simulink model "Progetto_Gruppo21_IZ"  (R2024b)
settings: Solver=FixedStepDiscrete  StartTime=0.0  StopTime=300  FixedStep=0.5  RelTol=1e-3  EnableMultiTasking=on
(part 1 of 2)
settings Model: PacingRate=0.500000  Creator=angel  LastModifiedBy=angel
settings OptimizationCC: DefaultParameterBehavior=Inlined  EnhancedBackFolding=on  PassReuseOutputArgsAs=Individual arguments  ZeroExternalMemoryAtStartup=off  ZeroInternalMemoryAtStartup=off  MaxStackSize=512  OptimizeBlockOrder=speed  DifferentSizesBufferReuse=on  OptimizationCustomize=off  EfficientTunableParamExpr=on
settings DebuggingCC: ParameterTunabilityLossMsg=error
settings HardwareCC: ProdBitPerPointer=32  ProdBitPerSizeT=32  ProdBitPerPtrDiffT=32  ProdLargestAtomicInteger=Long  ProdLargestAtomicFloat=Double  ProdWordSize=32  ProdLongLongMode=on  ProdHWDeviceType=ARM Compatible->ARM Cortex-M
settings RTWCC: Description=Embedded Coder  SystemTargetFile=ert.tlc  HardwareBoard=STM32G4xx Based  TemplateMakefile=ert_default_tmf  Toolchain=GNU Tools for ARM Embedded Processors
settings CodeAppCC: ForceParamTrailComments=on  IgnoreCustomStorageClasses=off  OperatorAnnotations=on  SimulinkDataObjDesc=on  SFDataObjDesc=on  InsertBlockDesc=on
settings ERTTargetCC: TargetLangStandard=C99 (ISO)  CodeReplacementLibrary=ARM Cortex-M  SupportVariableSizeSignals=on  ExtModeTransport=3  ExtModeStaticAlloc=on  ExtModeStaticAllocSize=2048  ExtModeMexFile=ext_xcp  ExtModeIntrfLevel=Level2 - Open

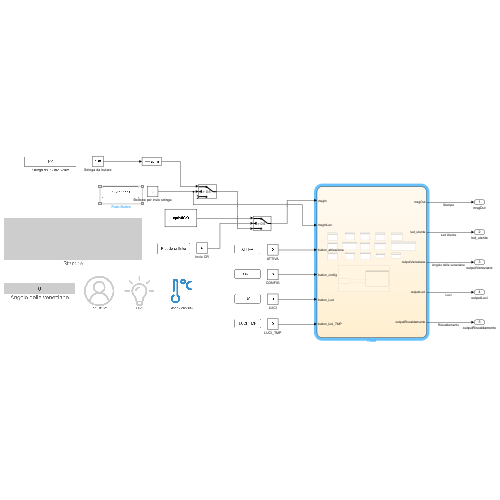
[thumbnail: Simulink's stored preview of the top-level diagram]
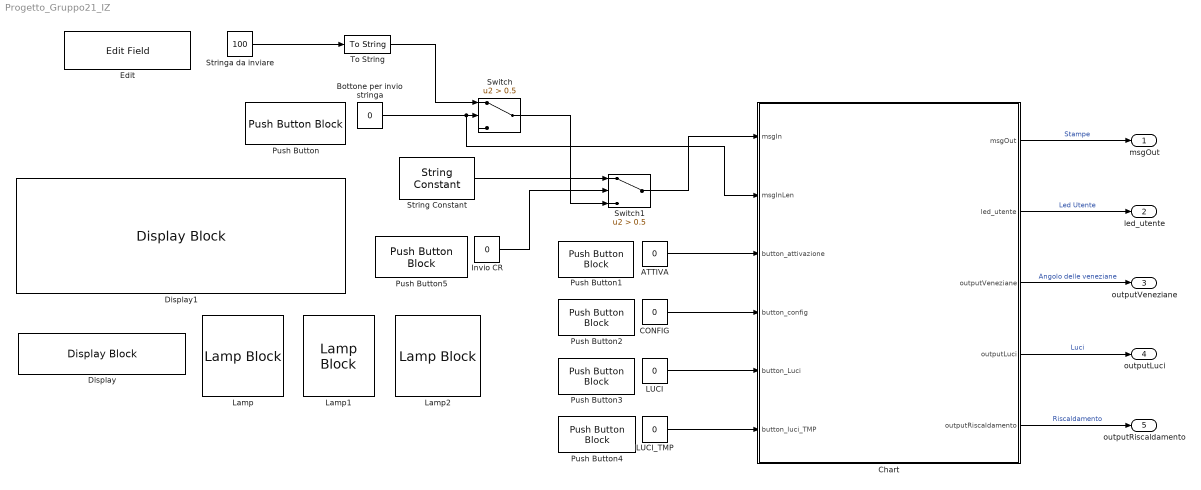
== system Progetto_Gruppo21_IZ ==
  ATTIVA : Constant  Value=0
  Bottone per invio stringa : Constant  Value=0
  CONFIG : Constant  Value=0
  Chart : Stateflow chart  TreatAsAtomicUnit=on
  Display : DisplayBlock  LabelPosition=Bottom  Transparency=1
  Display1 : DisplayBlock  LabelPosition=Bottom  Alignment=Left  Transparency=1
  Edit : EditField  LabelPosition=Bottom  ShowInitialText=on  Alignment=Center
  Invio CR : Constant  Value=0
  LUCI : Constant  Value=0
  LUCI_TMP : Constant  Value=0
  Lamp : LampBlock  LabelPosition=Bottom  Icon=Custom  CustomIcon=data:image/svg+xml;base64,CjwhLS0gR2VuZXJhdG9yOiB2aXNpb25jb3J0ZXggVlRyYWNlciAwLjYuNCAtLT4KPHN2ZyB2ZXJzaW9uPSIxLjEiIHhtbG5zPSJodHRwOi8vd3d3LnczLm9yZy8yMDAwL3N2ZyIgdmlld0JveD0iMCAwIDUxMiA1MTIiIHByZXNlcnZlQXNwZWN0UmF0aW89InhNaWRZTWlkIG1lZXQiPgo8cGF0aCBkPSJNMCAwIEMwLjk2NyAwLjAwMiAxLjkzNSAwLjAwNCAyLjkzMSAwLjAwNiBDMTcuMjY0IDAuMDUxIDMxLjIxIDAuNTYgNDUuMzEyIDMuMzEyIEM0Ni42NTggMy41NTQgNDYuNjU4IDMuNTU0IDQ4LjAzMSAzLjggQzk2LjcxOCAxMi42 ...(+8728 chars)
  Lamp1 : LampBlock  LabelPosition=Bottom  Icon=Custom  CustomIcon=data:image/svg+xml;base64,CjwhLS0gR2VuZXJhdG9yOiB2aXNpb25jb3J0ZXggVlRyYWNlciAwLjYuNCAtLT4KPHN2ZyB2ZXJzaW9uPSIxLjEiIHhtbG5zPSJodHRwOi8vd3d3LnczLm9yZy8yMDAwL3N2ZyIgdmlld0JveD0iMCAwIDUxMiA1MTIiIHByZXNlcnZlQXNwZWN0UmF0aW89InhNaWRZTWlkIG1lZXQiPgo8cGF0aCBkPSJNMCAwIEMwLjY2NSAwLjE4MiAxLjMzMSAwLjM2NCAyLjAxNyAwLjU1MSBDMjQuMjc0IDYuNzU2IDQzLjIzNiAxOS40MzkgNjAgMzUgQzYwLjY1NiAzNS41NzkgNjEuMzEyIDM2LjE1OCA2MS45ODggMzYuNzU0IEM4Mi4yNjEgNTUu ...(+12092 chars)
  Lamp2 : LampBlock  LabelPosition=Bottom  Icon=Custom  CustomIcon=data:image/svg+xml;base64,CjwhLS0gR2VuZXJhdG9yOiB2aXNpb25jb3J0ZXggVlRyYWNlciAwLjYuNCAtLT4KPHN2ZyB2ZXJzaW9uPSIxLjEiIHhtbG5zPSJodHRwOi8vd3d3LnczLm9yZy8yMDAwL3N2ZyIgdmlld0JveD0iMCAwIDUxMiA1MTIiIHByZXNlcnZlQXNwZWN0UmF0aW89InhNaWRZTWlkIG1lZXQiPgo8cGF0aCBkPSJNMCAwIEMxLjM2NCAwLjk4NiAyLjcyIDEuOTg1IDQuMDYyIDMgQzQuOTQ5IDMuNjE5IDUuODM2IDQuMjM3IDYuNzUgNC44NzUgQzE0LjY1MyAxMi4xMzcgMjEuMzQ5IDIzLjMwNiAyMi4yNCAzNC4xNjIgQzIyLjMwMSAzNi42NTIg ...(+7508 chars)
  Push Button : PushButtonBlock  ButtonText=Invio Stringa  OffValue=0.000000
  Push Button1 : PushButtonBlock  ButtonText=ATTIVA  OffValue=0.000000
  Push Button2 : PushButtonBlock  ButtonText=CONFIG  OffValue=0.000000
  Push Button3 : PushButtonBlock  ButtonText=LUCI  OffValue=0.000000
  Push Button4 : PushButtonBlock  ButtonText=LUCI_TMP  OffValue=0.000000
  Push Button5 : PushButtonBlock  ButtonText=Pressione Enter  OffValue=0.000000
  String Constant : StringConstant  String=sprintf('\r')
  Stringa da inviare : Constant  Value=100  SampleTime=Inf
  Switch : Switch  Criteria=u2 > Threshold  Threshold=0.5  SaturateOnIntegerOverflow=off  InputSameDT=off
  Switch1 : Switch  Criteria=u2 > Threshold  Threshold=0.5  SaturateOnIntegerOverflow=off  InputSameDT=off
  To String : ToString
  msgOut : Outport
  led_utente : Outport  Port=2
  outputVeneziane : Outport  Port=3
  outputLuci : Outport  Port=4
  outputRiscaldamento : Outport  Port=5
  wires:
  To String/1 -> Switch/1
  Switch/1 -> Switch1/3
  Stringa da inviare/1 -> To String/1
  Switch1/1 -> Chart/1(msgIn)
  Chart/1(msgOut) -> msgOut/1  "Stampe"
  ATTIVA/1 -> Chart/3(button_attivazione)
  Chart/2(led_utente) -> led_utente/1  "Led Utente"
  Chart/3(outputVeneziane) -> outputVeneziane/1  "Angolo delle veneziane"
  Chart/4(outputLuci) -> outputLuci/1  "Luci"
  Chart/5(outputRiscaldamento) -> outputRiscaldamento/1  "Riscaldamento"
  CONFIG/1 -> Chart/4(button_config)
  LUCI/1 -> Chart/5(button_Luci)
  LUCI_TMP/1 -> Chart/6(button_luci_TMP)
  Invio CR/1 -> Switch1/2
  String Constant/1 -> Switch1/1
  Bottone per invio stringa/1 -> Chart/2(msgInLen), Switch/2
